simulink model "task_1_0"  (R2023a)
settings: Solver=VariableStepAuto  StartTime=0.0  StopTime=10.0  RelTol=1e-3
settings Model: Creator=user  LastModifiedBy=user

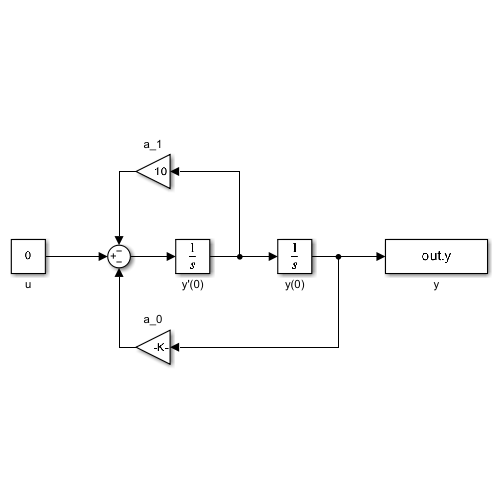
[thumbnail: Simulink's stored preview of the top-level diagram]
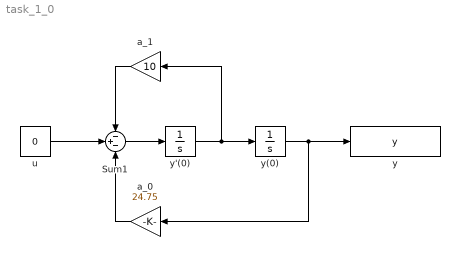
== system task_1_0 ==
  Sum1 : Sum  Inputs=-+-
  a_0 : Gain  Gain=24.75
  a_1 : Gain  Gain=10
  u : Constant  Value=0
  y : ToWorkspace  VariableName=y  SaveFormat=Timeseries  SampleTime=-1
  y'(0) : Integrator
  y(0) : Integrator  InitialCondition=1
  wires:
  u/1 -> Sum1/2
  Sum1/1 -> y'(0)/1
  y'(0)/1 -> a_1/1, y(0)/1
  y(0)/1 -> a_0/1, y/1
  a_0/1 -> Sum1/3
  a_1/1 -> Sum1/1
